simulink library "MCHP_Blockset"  (Simulink 7.5)
settings: Solver=ode45  SolverMode=SingleTasking  StartTime=0.0  StopTime=10.0  RelTol=1e-3
InitFcn:
  | disp('MCHP_Blockset_Library_InitFunction');
undefined symbols (not defined in the file): A0, A2, AD0, AVdd, B1, B5, B9, C10, C2, CMP2A, CMP3A, CMP4A, EXTREF1, EXTREF2, gcbh, MaxPer, MCHP_ACC_SAMx_Callback, MCHP_ADC_Callback, MCHP_ADC_HighSpeed_SAR_Callback, MCHP_ADC_HighSpeed_SAR_dsPIC_Callback, MCHP_ADC_SAME5x_Callback, MCHP_AFEC_SAM7x_Callback, MCHP_BUS_I2C_MASTER_callback, MCHP_BUS_SPI_callback, MCHP_C_function_Call_callback, MCHP_CN_Callback, MCHP_COMPARATOR1_callback, MCHP_CompilerOptimisation_Callback, MCHP_DACC_SAMx_Callback, MCHP_Digital_Input_Callback, MCHP_Digital_Output_Read_Callback, MCHP_Digital_Output_Write_Callback, MCHP_Fun, MCHP_HighSpeed_AnalogComparator_Callback, MCHP_IC_Callback, MCHP_IdleTask_Callback, MCHP_Interrupt_Callback, MCHP_Master_Callback, MCHP_MCPWM_Callback, MCHP_MCU_LOAD_Callback, MCHP_MCU_OVERLOAD_Callback, MCHP_MSI_Callback, MCHP_OC_HW_Callback, MCHP_OC_SW_Callback, MCHP_OP_AMP_Callback, MCHP_OrderInOut, MCHP_PDEC_Callback, MCHP_PGA_Callback, MCHP_PWM_Callback, MCHP_PWM_HighSpeed_Override_Callback, MCHP_PWM_HS_FEP_Callback, MCHP_PWM_SAM7x_Callback, MCHP_PWM_SAM7x_Override_Callback, MCHP_QDEC_SAMx_Callback, MCHP_QEI_Callback, MCHP_Scheduler_Options_Callback, MCHP_SECONDARY_CORE_Callback, MCHP_Tasks_State_Callback, MCHP_TCC_PWM_Callback, MCHP_TIMER_Config_Callback ... (+18)
libraries: MCHP_Blockset x2
(part 9 of 9)

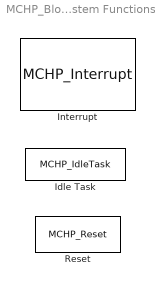
== system MCHP_Blockset/System Functions ==
  Idle Task : S-Function  InitFcn=MCHP_IdleTask_Callback(gcbh,'InitFcn');  FunctionName=MCHP_IdleTask  Parameters=-1,-1,-1,0  EnableBusSupport=off  mask(Idle Task (Call Simulink Subfunction)){MCHP_MASTERLINK=Dvpt_CN/Microchip Master}
      mask help:
      | The block output is a function call signal which must be connected to subsystem via the function call input port.
      |
      | Subsystem will be called iteratively within a never ending loop.
      | Simulink steps interrupt the Idle task execution.
      mask init:
      | MCHP_IdleTask_Callback(gcbh,'INITIALISATION');
      settings: PreSaveFcn=%MCHP_Fun.PreSaveFcn_DynamicOptions(gcbh);  OpenFcn=MCHP_IdleTask_Callback(gcbh,'OPEN');
      mask TabNameString: Main
      mask Display:
      | MCHP_DrawLogo;color('blue');fprintf('Idle Task');color('black');
      | port_label('output',1,'Fct');
  Interrupt : S-Function  InitFcn=MCHP_Interrupt_Callback(gcbh,'InitFcn');  FunctionName=MCHP_Interrupt  Parameters=-1,-1,-1,0,SS_ARCH,SS_ASYNCHRONOUS_INTERRUPT,SS_TIMESOURCE,SS_AsyncTimerRes,SS_AsyncTaskPriority  EnableBusSupport=off  mask(Interruption (Call Simulink Subfunction)){Interruption=Dynamic Options, Interruption_TXT=Not defined, InterruptionLongDesc=User Defined, IntPriority=6, IntPriority_Info=5, StartupExecute=off, Status=OK, MCHP_MASTERLINK=Dvpt_CN/Microchip Master, FPUNoSave=on, Triggered_Sub_TimeSource=is derived from model base rate, TrigsPeriod=0, TIMER_Resolution=Dynamic Options, TIMER_Resolution_TXT=0, MCHP_TIMER_REQUEST=0, MCHP_TIMER_RESULT=0, Info=0, SS_ASYNCHRONOUS_INTERRUPT=0, SS_TIMESOURCE=1, SS_AsyncTimerRes=-1, SS_AsyncTaskPriority=-1000, SS_ARCH=16}
      mask prompts: IntPriority "Interrupt Priority"; IntPriority_Info "Interrupt Priority"; StartupExecute "Force execution once at startup"; FPUNoSave "Do not save FPU context (triggered subsystep does not use floating point datatype)"; Triggered_Sub_TimeSource "Triggered subsystem Time source"; TrigsPeriod "Period for trigs (s)"; TIMER_Resolution "Resolution and max period"; Info "Timer Info:"
      mask help:
      | Only interruption defined by existing block can be used.
      |
      | The block output is a function call signal which must be connected to subsystem via the function call input port.
      mask init:
      | MCHP_Interrupt_Callback(gcbh,'INITIALISATION');
      settings: PreSaveFcn=MCHP_Fun.PreSaveFcn_DynamicOptions(gcbh);  OpenFcn=MCHP_Interrupt_Callback(gcbh,'OPEN');
      mask StyleString: popup(Dynamic Options),edit,edit,popup(0|1|2|3|4|5|6|7),popup(0|1|2|3|4|5|6|7),checkbox,edit,edit,checkbox,popup(is derived from model base rate|is derived from a hardware timer|is derived from trigs; trigs must be periodic),edit,popup(Dynamic Options),edit,edit,edit,edit,edit,edit,edit,edit,edit
      mask CallbackString: MCHP_Interrupt_Callback(gcbh,'DialogUpdate');|||||||||MCHP_Interrupt_Callback(gcbh,'DialogUpdate');|||||||||||
      mask TabNameString: Main,Main,Main,Main,Main,Main,Main,Main,Advanced,Advanced,Advanced,Advanced,Advanced,Advanced,Advanced,Advanced,Advanced,Advanced,Advanced,Advanced,Advanced
      mask Display:
      | MCHP_DrawLogo;color('blue');fprintf(['Interruption\n' get_param(gcbh,'InterruptionLongDesc')]);color('black');
      | port_label('output',1,'Fct');
  Reset : S-Function  FunctionName=MCHP_Reset  Parameters=SampleTime  EnableBusSupport=off  mask(UART Reset){SampleTime=-1, MCHP_MASTERLINK=UTestBoard_33FJ256GP710A_2/Microchip Master}
      mask prompts: SampleTime "Sample Time"
      mask help: Chip will reset when one elemnt of the input vecotr (or scalar) is different from 0.
      mask Display: MCHP_DrawLogo;fprintf('Reset');port_label('input',1,'rst' );

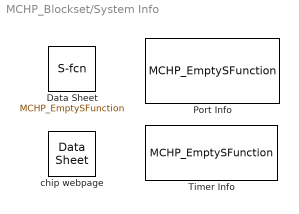
== system MCHP_Blockset/System Info ==
  Data Sheet : S-Function  FunctionName=MCHP_EmptySFunction  EnableBusSupport=off  mask{DOC_Type=datasheet, DOC_MCHP_Id=33FJ64MC802, DOC_FilePath=, DOC_FileLastCheckTime=[0 0 0 0 0 0], cpy_MCHP_Id=Undefined, MCHP_MASTERLINK=0}
      mask init:
      | MCHP_Doc_Callback(gcb,'INITIALISATION');
      settings: AttributesFormatString=%<cpy_MCHP_Id>  CopyFcn=MCHP_Doc_Callback(gcb,'COPY');  OpenFcn=MCHP_Doc_Callback(gcb,'OPEN');
      mask StyleString: popup(datasheet|errata|www),edit,edit,edit,edit,edit
      mask Display:
      | MCHP_DrawLogo;
      | plot([.8 0 0 1 1 .8 .8 1],[1 1 0 0 .8 1 .8 .8]);
      | text(.5,.6,'DOC','horizontalalignment','center');
      | text(.95,.05,'Pdf','verticalalignment','bottom','horizontalalignment','right');
  Port Info : S-Function  FunctionName=MCHP_EmptySFunction  EnableBusSupport=off  mask{MCHP_MASTERLINK=UTBoard_33EP12MC506_Comparator_OpAmps_ADC/Microchip Master}
      mask init:
      | MCHP_PortInfo_Callback(gcbh,'INITIALISATION');
      settings: CopyFcn=MCHP_PortInfo_Callback(gcb,'COPY');  OpenFcn=MCHP_PortInfo_Callback(gcb,'OPEN');
      mask Display: MCHP_DrawLogo;text(.05,0.5,'[Pin]  Port   -  Desc\n\n\n\n','verticalalignment','Middle','horizontalalignment','left');
  Timer Info : S-Function  FunctionName=MCHP_EmptySFunction  EnableBusSupport=off  mask{MCHP_MASTERLINK=Test_OC_HW/Microchip Master}
      mask init:
      | MCHP_TimerInfo_Callback(gcbh,'INITIALISATION');
      settings: CopyFcn=MCHP_TimerInfo_Callback(gcb,'COPY');  OpenFcn=MCHP_TimerInfo_Callback(gcb,'OPEN');
      mask Display: MCHP_DrawLogo;disp('3 timers used\n');
  chip webpage : MCHP_Blockset/System Info/Data Sheet  DOC_Type=www  DOC_MCHP_Id=33FJ64MC802  DOC_FileLastCheckTime=[0 0 0 0 0 0]  cpy_MCHP_Id=Undefined  MCHP_MASTERLINK=0
      settings: AttributesFormatString=%<cpy_MCHP_Id>

== system MCHP_Blockset/Timers ==
  TIMER Configuration : S-Function  InitFcn=MCHP_TIMER_Config_Callback(gcbh,'InitFcn');  FunctionName=MCHP_EmptySFunction  EnableBusSupport=off  mask(Timer Configuration){TIMER_Name=TimerA, TIMER_CustomName=pouet_p, TIMER_Ressource=Dynamic Options, TIMER_Ressource_TXT=No constraints [Prefered], TIMER_Ressource_Custom=[1], DoNotSetupChk=off, TIMER_PeriodChk=on, TIMER_Period=1e-5, TIMER_Resolution=Dynamic Options, TIMER_Resolution_TXT=Resol: 32(us)  -  MaxPer: 2.1(s), TIMER_Interrupt=off, TIMER_Use=Read only, TIMER_ShareChk=on, MCHP_TIMER_REQUEST={TimerA}{TmrCfg}20:1:1:0:[]:4194304;, MCHP_TIMER_RESULT=[2 65535 ], MCHP_USER_INTERRUPTS=, MCHP_MASTERLINK=Timer_Config_30f4011/Microchip Master, Info=Timer 2}
      mask prompts: TIMER_Name "Logical Timer Name"; TIMER_CustomName "Custom Logical Timer Name"; TIMER_Ressource "Timer Ressources"; TIMER_Ressource_TXT "Timer Ressources"; TIMER_Ressource_Custom "Timer List, example: [ 1  2  3  4  5 ]"; DoNotSetupChk "Do not setup Timer (preserve the timer for custom use)"; TIMER_PeriodChk "Period is set to its max value (65535)  ==>  0.0328(s)"; TIMER_Period "Set timer period (in seconds), max period is 0.0328(s)"; TIMER_Resolution "Resolution and max period"; TIMER_Interrupt "Define a user interrupt triggered by timer rollover"; TIMER_Use "Timer used for:"; TIMER_ShareChk "Others peripheral might use that timer (read operation only)"; Info "Timer info:"
      mask help:
      | Set Timer configuration
      | Peripheral that requrie a timer do not need this block. A timer is automatically assigned and configured in such case.
      mask init:
      | MCHP_TIMER_Config_Callback(gcbh,'INITIALISATION');
      settings: CopyFcn=MCHP_TIMER_Config_Callback(gcbh,'CopyFcn');  PreSaveFcn=MCHP_Fun.PreSaveFcn_DynamicOptions(gcbh);  OpenFcn=MCHP_TIMER_Config_Callback(gcbh,'OPEN');
      mask StyleString: popup(TimerA|TimerB|TimerC|TimerD|TimerE|TimerF|Custom Name),edit,popup(Dynamic Options),edit,edit,checkbox,checkbox,edit,popup(Dynamic Options),edit,checkbox,popup(Read only|Read / Write|Read / Write / Start - Stop / Period update),checkbox,edit,edit,edit,edit,edit
      mask CallbackString: MCHP_TIMER_Config_Callback(gcbh,'TIMER_Name');|MCHP_TIMER_Config_Callback(gcbh,'TIMER_CustomName');|MCHP_TIMER_Config_Callback(gcbh,'TIMER_Ressource');|||MCHP_TIMER_Config_Callback(gcbh,'DoNotSetupChk');|MCHP_TIMER_Config_Callback(gcbh,'TIMER_PeriodChk');||MCHP_TIMER_Config_Callback(gcbh,'TIMER_Resolution');|||MCHP_TIMER_Config_Callback(gcbh,'TIMER_Use');||||||
      mask Display: MCHP_DrawLogo;disp('TimerA\nConfiguration')

== system MCHP_Blockset/User Functions ==
  C Function Call : S-Function  FunctionName=MCHP_C_function_Call  Parameters=MCHP_C_function_Call_callback(gcbh,'S_INPUT'),MCHP_C_function_Call_callback(gcbh,'S_OUTPUT'),MCHP_C_function_Call_callback(gcbh,'S_INPUT_Size'),MCHP_C_function_Call_callback(gcbh,'S_OUTPUT_Size'),MCHP_C_function_Call_callback(gcbh,'S_ListCustomDatatype'),SampleTime,MCHP_OrderInOut(gcbh)  EnableBusSupport=off  mask(C Function Call){ParseFilesChkbx=off, ListFunctions1=Custom Function, Function1=extern void __delay_ms(unsigned long t_ms);, AddHeaderDeclaration=off, Function1Type=when block is updated (default), Fct1BlockIn=, FctReturnBlockOut=on, Fct1BlockOut=, DataCollected=0, ORDERING=None, SampleTime=-1, S_INPUT=0, S_INPUT_Size=0, S_OUTPUT=0, S_OUTPUT_Size=0, S_ListCustomDatatype=0, MCHP_CRC=0, MCHP_MASTERLINK=, PinDigitalInput=[], PinDigitalOutput=[], PinAnalogInput=[], MCHP_PORT=}
      mask prompts: ParseFilesChkbx "Parse user file to list functions available (need to re-open this block GUI)"; ListFunctions1 "Functions found:"; Function1 "Function Declaration:"; AddHeaderDeclaration "Add this function declaration in header file"; Function1Type "execute function:"; Fct1BlockIn "Block Input (coma separated function parameters)"; FctReturnBlockOut "Function returned value is a block output (return value must be a scalar or a struct)"; Fct1BlockOut "Block Output (coma separated function parameters)"; DataCollected "CollectedData"; ORDERING "Block execution ordering"; SampleTime "Sample Time"; PinDigitalInput "List of port used as Digital Input (like  A[1 2] B12 ...)"; PinDigitalOutput "List of port used as Digital Output (like  A[1 2] B12 ...)"; PinAnalogInput "List of port used as Analog Input (like  A[1 2] B12 ...)"
      mask init:
      | MCHP_C_function_Call_callback(gcbh,'INITIALISATION');
      settings: PreSaveFcn=set_param(gcbh,'ListFunctions1','Custom Function');  OpenFcn=MCHP_C_function_Call_callback(gcbh,'OPEN');
      mask StyleString: checkbox,popup(Custom Function),edit,checkbox,popup(when block is updated (default)|only once at power-up time),edit,checkbox,edit,edit,popup(None|Input|Output|Input & Output),edit,edit,edit,edit,edit,edit,edit,edit,edit,edit,edit,edit
      mask CallbackString: |MCHP_Fun.BlockUpdate(gcbh);||||||||||||||||||||
      mask TabNameString: Function,Function,Function,Function,Function,Function,Function,Function,Function,Function,Function,Function,Function,Function,Function,Function,Function,Function,Pins Configuration,Pins Configuration,Pins Configuration,Pins Configuration
      mask Display:
      | MCHP_DrawLogo;fprintf('C function\n__delay_ms');
      | port_label('input',1,'t_ms');

== system MCHP_Blockset/Digital IO/Digital Output ==
  In1 : Inport
  Digital Output Write : MCHP_Blockset/Digital IO/Digital Output Write  PORT=Dynamic Options  PORT_TXT="A   [ 0  1  2  3  4  5  6  7  9  10  14  15 ]"  PIN=0  PACK=off  SIMULTANEOUS=off  ORDERING=None  SampleTime=-1  MCHP_PORT={Digital Out}{DOU}1:1:A0;{Digital Out}{DOU}1:1:A1;{Digital Out}{DOU}1:1:A2;  MCHP_MASTERLINK=UTester_33EP512MU810_NewDigitOutBlock/Microchip Master
  wires:
  In1/1 -> Digital Output Write/1
